simulink model "gm_my_hdlcoder_sqrt_bitset_control"  (R2024a)
settings: Solver=VariableStepAuto  StartTime=0.0  StopTime=stoptime  RelTol=1e-3
libraries: dspsrcs4 x1
settings Model: Creator=lingg  LastModifiedBy=lingg
settings DataIOCC: SaveOutput=off  SignalLogging=off  SaveTime=off  ReturnWorkspaceOutputs=off
settings OptimizationCC: BlockReduction=off  ConditionallyExecuteInputs=off
settings DebuggingCC: InheritedTsInSrcMsg=none  IntegerOverflowMsg=none  IntegerSaturationMsg=none

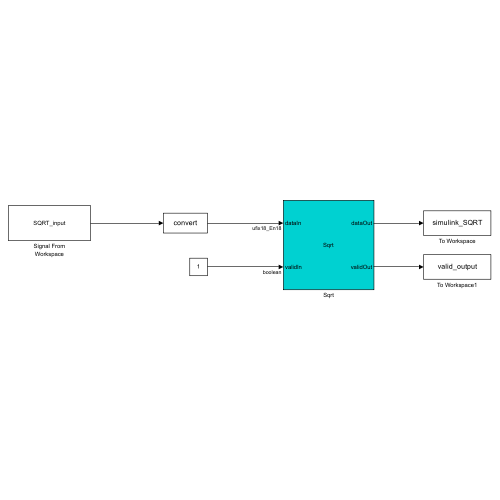
[thumbnail: Simulink's stored preview of the top-level diagram]
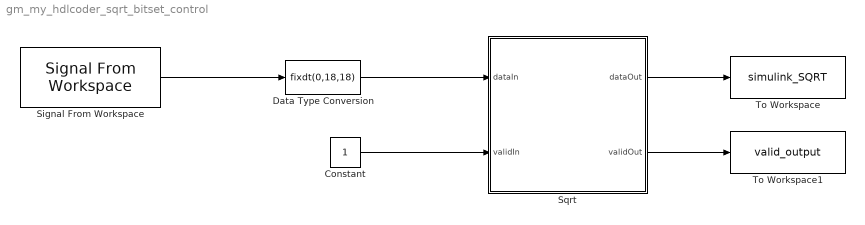
== system gm_my_hdlcoder_sqrt_bitset_control ==
  Constant : Constant  OutDataTypeStr=boolean  SampleTime=-1
  Data Type Conversion : DataTypeConversion  OutDataTypeStr=fixdt(0,18,18)  RndMeth=Floor
  Signal From Workspace : dspsrcs4/Signal From Workspace  X=SQRT_input  Ts=1  nsamps=1  OutputAfterFinalValue=Setting to zero  ignoreOrWarnInputAndFrameLengths=off  OutputFrames=off
  Sqrt : Subsystem  mask(Sqrt){latencyMode=Max, customLatencyValue=double(0), OutDataTypeStr=Inherit: Same as first input, SaturateOnIntegerOverflow='on', RndMeth=Floor}
      mask prompts: latencyMode "Latency strategy"; customLatencyValue "Custom latency"; OutDataTypeStr "Output data type:"; SaturateOnIntegerOverflow "Simulink:blkprm_prompts:AllBlksSaturate"; RndMeth "Integer rounding mode:"
      mask help: Sqrt block with control ports and simulates with latency
      mask init:
      | OutDataTypeStr = 'Inherit: Same as first input';
      | RndMeth = double(3);
      | SaturateOnIntegerOverflow = 'on';
      | curr_blk_name = 'my_hdlcoder_sqrt_bitset_control/Sqrt';
      | customLatencyValue = double(0);
      | latencyMode = double(1);
      | sys_name = 'my_hdlcoder_sqrt_bitset_control';
      mask Help: helpview(fullfile(docroot,'hdlcoder','helptargets.map'),'HDL_Math_Sqrtfcn');
      mask TypeOptions latencyMode: Max | Min | Custom | Zero
      mask Callback latencyMode:
      | lat = get_param(gcb,'latencyMode');
      | if(strcmpi(lat,'Custom'))
      |     set_param(gcb,'MaskEnables',{'on','on','on','on','on'});
      | else
      |     set_param(gcb,'MaskEnables',{'on','off','on','on','on'});
      | end
      mask TypeOptions RndMeth: Zero | Ceiling | Floor | Nearest | Simplest
      mask Display:
      | disp('Sqrt')
      | port_label('input', 1, 'dataIn')
      | port_label('output', 1, 'dataOut')
      | port_label('input', 2, 'validIn')
      | port_label('output', 2, 'validOut')
  To Workspace : ToWorkspace  VariableName=simulink_SQRT  SampleTime=-1
      settings: Save2DSignal=2-D array (concatenate along first dimension)
  To Workspace1 : ToWorkspace  VariableName=valid_output  SampleTime=-1
      settings: Save2DSignal=2-D array (concatenate along first dimension)
  wires:
  Sqrt/2(validOut) -> To Workspace1/1
  Sqrt/1(dataOut) -> To Workspace/1
  Constant/1 -> Sqrt/2(validIn)
  Data Type Conversion/1 -> Sqrt/1(dataIn)
  Signal From Workspace/1 -> Data Type Conversion/1

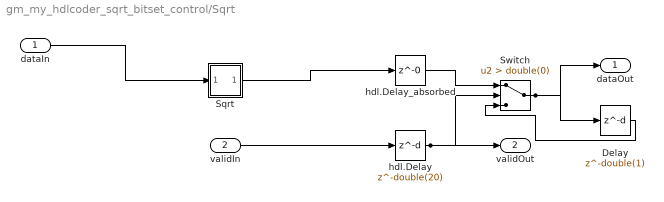
== system gm_my_hdlcoder_sqrt_bitset_control/Sqrt ==
  dataIn : Inport  OutDataTypeStr=fixdt(0, 18, 18)  SampleTime=1
  validIn : Inport  Port=2  OutDataTypeStr=boolean  SampleTime=1
  Delay : Delay  DelayLength=double(1)  InitialCondition=0  SampleTime=1
  Sqrt : Subsystem
  Switch : Switch  Criteria=u2 > Threshold  Threshold=double(0)  OutDataTypeStr=fixdt(0, 18, 18)  SampleTime=1  SaturateOnIntegerOverflow=off  InputSameDT=off
  hdl.Delay : Delay  DelayLength=double(20)  InitialCondition=0  SampleTime=1
  hdl.Delay_absorbed : Delay  DelayLength=0
  dataOut : Outport  SampleTime=1
  validOut : Outport  Port=2  SampleTime=1
  wires:
  dataIn/1 -> Sqrt/1(In1)
  validIn/1 -> hdl.Delay/1
  Switch/1 -> dataOut/1, Delay/1
  hdl.Delay/1 -> validOut/1, Switch/2
  Delay/1 -> Switch/3
  hdl.Delay_absorbed/1 -> Switch/1
  Sqrt/1(Out1) -> hdl.Delay_absorbed/1

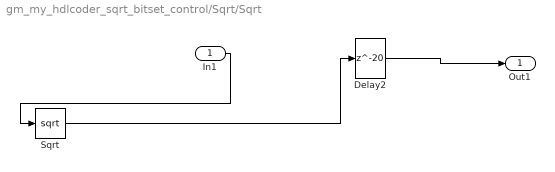
== system gm_my_hdlcoder_sqrt_bitset_control/Sqrt/Sqrt ==
  In1 : Inport
  Delay2 : Delay  DelayLength=20
  Sqrt : Sqrt
  Out1 : Outport
  wires:
  In1/1 -> Sqrt/1
  Sqrt/1 -> Delay2/1
  Delay2/1 -> Out1/1
